simulink model "VTOL_v2_MW"  (R2018b)
settings: Solver=FixedStepAuto  StartTime=0.0  StopTime=inf  FixedStep=Ts  RelTol=1e-3  EnableMultiTasking=on
values from neighbouring files (symbols this model uses):
  Ts = 1/100    (= 0.01)    [VTOL_params.m]
undefined symbols (not defined in the file or in its folder): color, deltaprops, dev, led_mask, Main, mode, MRC, pwm_output0
libraries: aerolibutil x7, px4uORBlib x6, pwm_sig_converters x4, px4Sensorslib x3, simulink x3, px4lib x1, sharedtransform x1
(part 2 of 2)

== matlab function VTOL_v2_MW/PX4 SD Card Logger4/SDCard_logger ==
  data: en input boolean; data input; logname parameter uint8; cacheflag parameter boolean; numRecs parameter uint32
%% PX4 SD Card Logger
% Note: All data needs to be of the same type (e.g. double)
% Header information format:
%           String "MWLOG"
%           Time/Date 4 bytes (time())
%           Number of Signals per record Logged 1 byte (256 max)
%           Data Type of Signals Logged  1 byte (1-10)
%           Number of bytes per record 2 bytes (65535 max)
% This does NOT include the number of data sets logged.
% i.e. The Reader is responsible for reading until EOF.
% Steve Kuznicki
% Copyright 2018 The MathWorks, Inc.

function SDCard_logger(en, data, logname, cacheflag, numRecs)

persistent fp count elem_size vect_size datastore timestore count_prev

if coder.target('Rtw')
    
    coder.cinclude('<stdio.h>');
    coder.cinclude('<time.h>');
    
    if coder.target('Rtw')
        coder.cinclude('<drivers/drv_hrt.h>');
    end
    
    if coder.target('Rtw')
        timestamp=coder.opaque('uint64_t');
        timestamp=coder.ceval('hrt_absolute_time');
    else
        timestamp = uint64(0);
    end
    
    if isempty(count)
        count = uint32(0);
        count_prev=count;
        fp = coder.opaque('FILE*', 'NULL');
        if cacheflag == true
            datastore = zeros(numRecs*uint32(coder.const(numel(data))), 1, 'like', data);
            timestore=uint64(zeros(numRecs, 1));
        end
        
        [elsize, eltype] = get_elem_size(data);
        elem_size = coder.const(uint16(elsize));
        elem_type = coder.const(uint8(eltype));
        vect_size = coder.const(uint8(numel(data)));
        coder.ceval('printf',['OPENING file %s vect_size %d elem_size %d numRecs %d %c' uint8(0)], ...
            [logname,'.bin', int8(0)], uint32(vect_size), uint32(elem_size), uint32(numRecs), uint8(10));
        fp = coder.ceval('fopen', [logname,'.bin', int8(0)], ['wb', int8(0)]);
        
        % Write header information here
        % header token + version
        mlStrVer = 'MWLOG';
        coder.ceval('fwrite', coder.rref(mlStrVer), uint32(1), length(mlStrVer), fp);
        % date/time
        tm = uint32(0);
        tmptr = uint32(0);
        tm = coder.ceval('time',coder.wref(tmptr));
        coder.ceval('fwrite', coder.rref(tm), uint32(4), uint32(1), fp);
        % number of elements in each record
        coder.ceval('fwrite', coder.rref(vect_size), uint32(1), uint32(1), fp);
        % data type of the elements
        coder.ceval('fwrite', coder.rref(elem_type), uint32(1), uint32(1), fp);
        % size of each record in bytes
        recSize = elem_size * uint16(vect_size);
        coder.ceval('fwrite', coder.rref(recSize), uint32(2), uint32(1), fp);
        coder.ceval('fclose', fp);
    end
    
    
    if (en && (count < numRecs))
              
        % cache data in memory or use fwrite
        if cacheflag == true
            addr = (count*uint32(vect_size))+1;
            for idx = 1:vect_size
                datastore(addr) = data(idx);
                addr = addr + 1;
            end
            timestore(count+uint32(1))=uint64(timestamp);
        else
            % open file in append mode
            fp = coder.ceval('fopen', [logname,'.bin', int8(0)], ['ab', int8(0)]);
            coder.ceval('fwrite', coder.rref(data), elem_size, vect_size, fp);
            if coder.target('Rtw')
                coder.ceval('fwrite', coder.rref(timestamp), uint32(8), uint32(1), fp);
            end
            coder.ceval('fflush', fp);
            coder.ceval('fclose', fp);
        end
        count = count + uint32(1);
        
    else
        
        if cacheflag
            % open file in append mode
            fp = coder.ceval('fopen', [logname,'.bin', int8(0)], ['ab', int8(0)]);
            coder.ceval('printf',['CLOSING file. count = %d %c' uint8(0)], uint32(count), uint8(10));
            for idx=count_prev+1:count
                for idx2=(idx-1)*double(vect_size)+1:(idx-1)*double(vect_size)+double(vect_size)
                    coder.ceval('fwrite', coder.rref(datastore(idx2)), elem_size, uint32(1), fp);
                end
                coder.ceval('fwrite', coder.rref(timestore(idx)), uint32(8), uint32(1), fp);
            end
            coder.ceval('fflush', fp);
            coder.ceval('fclose', fp);
        end
        count_prev=count;
    end
end

% return the size of the element in bytes
    function [elem_size, dtype] = get_elem_size(data)
        switch(class(data))
            case 'double'
                elem_size = 8;
                dtype = 1;
            case 'single'
                elem_size = 4;
                dtype = 2;
            case 'int32'
                elem_size = 4;
                dtype = 3;
            case 'uint32'
                elem_size = 4;
                dtype = 4;
            case 'int16'
                elem_size = 2;
                dtype = 5;
            case 'uint16'
                elem_size = 2;
                dtype = 6;
            case 'int8'
                elem_size = 1;
                dtype = 7;
            case 'uint8'
                elem_size = 1;
                dtype = 8;
            case 'logical'
                elem_size = 1;
                dtype = 9;
            case 'embedded.fi'
                nt = numerictype(data);
                elem_size = 2^ceil(log2(ceil(nt.WordLength / 8)));
                dtype = 10;
        end
        if ~isreal(data)
            elem_size = elem_size*2;
        end
        
        elem_size = uint16(elem_size);
        dtype = uint8(dtype);
    end
end

== matlab function VTOL_v2_MW/MATLAB Function12 ==
  data: sticks input; q_ref output; offset_stick input
function q_ref = sticks2quat(sticks, offset_stick)

persistent ail;
persistent ele;
persistent rud;
persistent S2;
if isempty(ail)
    ail = single(0);
end
if isempty(ele)
    ele = single(0);
end
if isempty(rud)
    rud = single(0);
end
if isempty(S2)
    S2 = single(0);
end

offset = 0;

SB = sticks(5); % MOde selector
if SB < -0.1
    % mode hover stable
    %thrust = sticks(1);
    ail = 1.5*sticks(2);
    ele = 1.5*sticks(3);
    rud = 1.5*sticks(4);
    
%elseif SB < 0.1
%    % Not used now
else
    % Mode servo setting quat, acro?
    S2 = 0.05*(sticks(6)+1); % Sensitivity setting
    ail = ail + S2*sticks(2);
    ele = ele + S2*sticks(3);
    rud = rud + S2*sticks(4);
    
end

%ElevonL = -ail-ele;
%ElevonR = -ail+ele;
%ThrustL = thrust+rud;
%ThrustR = thrust-rud;
%{
q_init = [cos(pi/4), 0, sin(pi/4), 0];
qyaw = [q00 0 0 q03];
qpitch = [q10 0 q12 0];
qroll = [q20 q21 0 0];
q0 = quatmultiply(q_init,qyaw)
q1 = quatmultiply(q0, qpitch);
q_ref = quatmultiply(q1,qroll)'
%}

%offset = 0; %deg2rad(5); % set on elevons instead
SA = sticks(7);
if SA < -0.1 % point up for hover
    q_init = [cos((pi/4 + offset)), 0, sin((pi/4 + offset)), 0];
elseif SA < 0.1 % Point forward for flight
    q_init = [cos((pi/20 + offset)), 0, sin((pi/20 + offset)), 0];
else % Point backwards for upsidedown flying
    q_init = [cos((pi/2 + offset)), 0, sin((pi/2 + offset)), 0];
end

q00 = cos(rud/2);
q03 = sin(rud/2);
q10 = cos(-ele/2);
q12 = sin(-ele/2);
q20 = cos(ail/2);
q21 = sin(ail/2);


qyaw = [q00 0 0 q03];
qpitch = [q10 0 q12 0];
qroll = [q20 q21 0 0];

%{
q0 = quatmultiply(qyaw,qpitch);
q1 = quatmultiply(q0, qroll);
q_ref = quatmultiply(q1,q_init)';
 %}
q0 = quatmultiply(q_init, qyaw);
q1 = quatmultiply(q0, qpitch);
q_ref = quatmultiply(q1,qroll)';

== matlab function VTOL_v2_MW/PX4 SD Card Logger1/SDCard_logger ==
  data: en input boolean; data input; logname parameter uint8; cacheflag parameter boolean; numRecs parameter uint32
%% PX4 SD Card Logger
% Note: All data needs to be of the same type (e.g. double)
% Header information format:
%           String "MWLOG"
%           Time/Date 4 bytes (time())
%           Number of Signals per record Logged 1 byte (256 max)
%           Data Type of Signals Logged  1 byte (1-10)
%           Number of bytes per record 2 bytes (65535 max)
% This does NOT include the number of data sets logged.
% i.e. The Reader is responsible for reading until EOF.
% Steve Kuznicki
% Copyright 2018 The MathWorks, Inc.

function SDCard_logger(en, data, logname, cacheflag, numRecs)

persistent fp count elem_size vect_size datastore timestore count_prev

if coder.target('Rtw')
    
    coder.cinclude('<stdio.h>');
    coder.cinclude('<time.h>');
    
    if coder.target('Rtw')
        coder.cinclude('<drivers/drv_hrt.h>');
    end
    
    if coder.target('Rtw')
        timestamp=coder.opaque('uint64_t');
        timestamp=coder.ceval('hrt_absolute_time');
    else
        timestamp = uint64(0);
    end
    
    if isempty(count)
        count = uint32(0);
        count_prev=count;
        fp = coder.opaque('FILE*', 'NULL');
        if cacheflag == true
            datastore = zeros(numRecs*uint32(coder.const(numel(data))), 1, 'like', data);
            timestore=uint64(zeros(numRecs, 1));
        end
        
        [elsize, eltype] = get_elem_size(data);
        elem_size = coder.const(uint16(elsize));
        elem_type = coder.const(uint8(eltype));
        vect_size = coder.const(uint8(numel(data)));
        coder.ceval('printf',['OPENING file %s vect_size %d elem_size %d numRecs %d %c' uint8(0)], ...
            [logname,'.bin', int8(0)], uint32(vect_size), uint32(elem_size), uint32(numRecs), uint8(10));
        fp = coder.ceval('fopen', [logname,'.bin', int8(0)], ['wb', int8(0)]);
        
        % Write header information here
        % header token + version
        mlStrVer = 'MWLOG';
        coder.ceval('fwrite', coder.rref(mlStrVer), uint32(1), length(mlStrVer), fp);
        % date/time
        tm = uint32(0);
        tmptr = uint32(0);
        tm = coder.ceval('time',coder.wref(tmptr));
        coder.ceval('fwrite', coder.rref(tm), uint32(4), uint32(1), fp);
        % number of elements in each record
        coder.ceval('fwrite', coder.rref(vect_size), uint32(1), uint32(1), fp);
        % data type of the elements
        coder.ceval('fwrite', coder.rref(elem_type), uint32(1), uint32(1), fp);
        % size of each record in bytes
        recSize = elem_size * uint16(vect_size);
        coder.ceval('fwrite', coder.rref(recSize), uint32(2), uint32(1), fp);
        coder.ceval('fclose', fp);
    end
    
    
    if (en && (count < numRecs))
              
        % cache data in memory or use fwrite
        if cacheflag == true
            addr = (count*uint32(vect_size))+1;
            for idx = 1:vect_size
                datastore(addr) = data(idx);
                addr = addr + 1;
            end
            timestore(count+uint32(1))=uint64(timestamp);
        else
            % open file in append mode
            fp = coder.ceval('fopen', [logname,'.bin', int8(0)], ['ab', int8(0)]);
            coder.ceval('fwrite', coder.rref(data), elem_size, vect_size, fp);
            if coder.target('Rtw')
                coder.ceval('fwrite', coder.rref(timestamp), uint32(8), uint32(1), fp);
            end
            coder.ceval('fflush', fp);
            coder.ceval('fclose', fp);
        end
        count = count + uint32(1);
        
   else
        
        if cacheflag
            % open file in append mode
            fp = coder.ceval('fopen', [logname,'.bin', int8(0)], ['ab', int8(0)]);
            coder.ceval('printf',['CLOSING file. count = %d %c' uint8(0)], uint32(count), uint8(10));
            for idx=count_prev+1:count
                for idx2=(idx-1)*double(vect_size)+1:(idx-1)*double(vect_size)+double(vect_size)
                    coder.ceval('fwrite', coder.rref(datastore(idx2)), elem_size, uint32(1), fp);
                end
                coder.ceval('fwrite', coder.rref(timestore(idx)), uint32(8), uint32(1), fp);
            end
            coder.ceval('fflush', fp);
            coder.ceval('fclose', fp);
        end
        count_prev=count;
    end
end

% return the size of the element in bytes
    function [elem_size, dtype] = get_elem_size(data)
        switch(class(data))
            case 'double'
                elem_size = 8;
                dtype = 1;
            case 'single'
                elem_size = 4;
                dtype = 2;
            case 'int32'
                elem_size = 4;
                dtype = 3;
            case 'uint32'
                elem_size = 4;
                dtype = 4;
            case 'int16'
                elem_size = 2;
                dtype = 5;
            case 'uint16'
                elem_size = 2;
                dtype = 6;
            case 'int8'
                elem_size = 1;
                dtype = 7;
            case 'uint8'
                elem_size = 1;
                dtype = 8;
            case 'logical'
                elem_size = 1;
                dtype = 9;
            case 'embedded.fi'
                nt = numerictype(data);
                elem_size = 2^ceil(log2(ceil(nt.WordLength / 8)));
                dtype = 10;
        end
        if ~isreal(data)
            elem_size = elem_size*2;
        end
        
        elem_size = uint16(elem_size);
        dtype = uint8(dtype);
    end
end

== matlab function VTOL_v2_MW/Subsystem/MATLAB Function14 ==
  data: target_altitude output single; throttle input single; init_alt input single
function target_altitude = fcn(throttle, init_alt)

persistent target_alt;
if isempty(target_alt)
    target_alt = init_alt;
end

target_alt = target_alt + 0.005*throttle;
target_altitude = target_alt;

== matlab function VTOL_v2_MW/MATLAB Function14 ==
  data: tao input; u_deltaL output; u_omegaL input; u_omegaR input; v input; u_deltaR output
function [u_deltaL, u_deltaR] = torqueConverter(tao, u_omegaL, u_omegaR, v)

KV = 1300;
V = 3.7*3;
loadFactor = 0.5;
maxRPM = KV*V*loadFactor;

omegaL = maxRPM*0.5*(u_omegaL+1); % Shift from [-1,1] to [0,1]
omegaR = maxRPM*0.5*(u_omegaR+1);
k1 = 0;
k2 = 2.41e-6;
k3 = 0;
k4 = 4.06e-6;

% These functons are derived in my paper, see
% https://github.com/Trobolit/MastersThesis/blob/master/thesis/main.pdf
u_deltaL = -0.5*tao(2)/(k1*sign(v(1))*sum(v.^2) + k2*omegaL^2) ...
           - 0.5*tao(1)/(k3*sign(v(1))*sum(v.^2) + k4*omegaL^2);

u_deltaR = -0.5*tao(2)/(k1*sign(v(1))*sum(v.^2) + k2*omegaR^2) ...
           + 0.5*tao(1)/(k3*sign(v(1))*sum(v.^2) + k4*omegaR^2);

== matlab function VTOL_v2_MW/MATLAB Function11 ==
  data: P input; D input; axisgains input; angErr input; taos output; w input
function taos = taos_fordecoupler(P, D, axisgains,angErr, w)

taos = single([0;0;0]);

%P1 = 1; %30; %1
%P2 = 0.5; %7.5; %0.25
cx = axisgains(1);%10;
cy = axisgains(2);%100;
cz = axisgains(3);%1;


% Emil Fresk P2 controller
taos = -P.*angErr - D.*w;
% Adjustment for actuators
taos(1) = cx*taos(1);
taos(2) = cy*taos(2);
taos(3) = cz*taos(3);

== matlab function VTOL_v2_MW/MATLAB Function15 ==
  data: voltage input single; stopsig output uint16; cutoff input single
function stopsig = fcn(voltage, cutoff)

if voltage<cutoff
    stopsig = uint16(2000);
else
    stopsig = uint16(1000);
end

== matlab function VTOL_v2_MW/MATLAB Function16 ==
  data: offset_stick input; offset output
function offset = fcn(offset_stick)

offset = single(offset_stick);
% Shift to center
offset = offset-1500;
% Range is ~1000-2000, ie +-500, but in is +-1
offset = 0.5*offset./500 + 0.75;

== matlab function VTOL_v2_MW/PX4 SD Card Logger3/SDCard_logger ==
  data: en input boolean; data input; logname parameter uint8; cacheflag parameter boolean; numRecs parameter uint32
%% PX4 SD Card Logger
% Note: All data needs to be of the same type (e.g. double)
% Header information format:
%           String "MWLOG"
%           Time/Date 4 bytes (time())
%           Number of Signals per record Logged 1 byte (256 max)
%           Data Type of Signals Logged  1 byte (1-10)
%           Number of bytes per record 2 bytes (65535 max)
% This does NOT include the number of data sets logged.
% i.e. The Reader is responsible for reading until EOF.
% Steve Kuznicki
% Copyright 2018 The MathWorks, Inc.

function SDCard_logger(en, data, logname, cacheflag, numRecs)

persistent fp count elem_size vect_size datastore timestore count_prev

if coder.target('Rtw')
    
    coder.cinclude('<stdio.h>');
    coder.cinclude('<time.h>');
    
    if coder.target('Rtw')
        coder.cinclude('<drivers/drv_hrt.h>');
    end
    
    if coder.target('Rtw')
        timestamp=coder.opaque('uint64_t');
        timestamp=coder.ceval('hrt_absolute_time');
    else
        timestamp = uint64(0);
    end
    
    if isempty(count)
        count = uint32(0);
        count_prev=count;
        fp = coder.opaque('FILE*', 'NULL');
        if cacheflag == true
            datastore = zeros(numRecs*uint32(coder.const(numel(data))), 1, 'like', data);
            timestore=uint64(zeros(numRecs, 1));
        end
        
        [elsize, eltype] = get_elem_size(data);
        elem_size = coder.const(uint16(elsize));
        elem_type = coder.const(uint8(eltype));
        vect_size = coder.const(uint8(numel(data)));
        coder.ceval('printf',['OPENING file %s vect_size %d elem_size %d numRecs %d %c' uint8(0)], ...
            [logname,'.bin', int8(0)], uint32(vect_size), uint32(elem_size), uint32(numRecs), uint8(10));
        fp = coder.ceval('fopen', [logname,'.bin', int8(0)], ['wb', int8(0)]);
        
        % Write header information here
        % header token + version
        mlStrVer = 'MWLOG';
        coder.ceval('fwrite', coder.rref(mlStrVer), uint32(1), length(mlStrVer), fp);
        % date/time
        tm = uint32(0);
        tmptr = uint32(0);
        tm = coder.ceval('time',coder.wref(tmptr));
        coder.ceval('fwrite', coder.rref(tm), uint32(4), uint32(1), fp);
        % number of elements in each record
        coder.ceval('fwrite', coder.rref(vect_size), uint32(1), uint32(1), fp);
        % data type of the elements
        coder.ceval('fwrite', coder.rref(elem_type), uint32(1), uint32(1), fp);
        % size of each record in bytes
        recSize = elem_size * uint16(vect_size);
        coder.ceval('fwrite', coder.rref(recSize), uint32(2), uint32(1), fp);
        coder.ceval('fclose', fp);
    end
    
    
    if (en && (count < numRecs))
              
        % cache data in memory or use fwrite
        if cacheflag == true
            addr = (count*uint32(vect_size))+1;
            for idx = 1:vect_size
                datastore(addr) = data(idx);
                addr = addr + 1;
            end
            timestore(count+uint32(1))=uint64(timestamp);
        else
            % open file in append mode
            fp = coder.ceval('fopen', [logname,'.bin', int8(0)], ['ab', int8(0)]);
            coder.ceval('fwrite', coder.rref(data), elem_size, vect_size, fp);
            if coder.target('Rtw')
                coder.ceval('fwrite', coder.rref(timestamp), uint32(8), uint32(1), fp);
            end
            coder.ceval('fflush', fp);
            coder.ceval('fclose', fp);
        end
        count = count + uint32(1);
        
    else
        
        if cacheflag
            % open file in append mode
            fp = coder.ceval('fopen', [logname,'.bin', int8(0)], ['ab', int8(0)]);
            coder.ceval('printf',['CLOSING file. count = %d %c' uint8(0)], uint32(count), uint8(10));
            for idx=count_prev+1:count
                for idx2=(idx-1)*double(vect_size)+1:(idx-1)*double(vect_size)+double(vect_size)
                    coder.ceval('fwrite', coder.rref(datastore(idx2)), elem_size, uint32(1), fp);
                end
                coder.ceval('fwrite', coder.rref(timestore(idx)), uint32(8), uint32(1), fp);
            end
            coder.ceval('fflush', fp);
            coder.ceval('fclose', fp);
        end
        count_prev=count;
    end
end

% return the size of the element in bytes
    function [elem_size, dtype] = get_elem_size(data)
        switch(class(data))
            case 'double'
                elem_size = 8;
                dtype = 1;
            case 'single'
                elem_size = 4;
                dtype = 2;
            case 'int32'
                elem_size = 4;
                dtype = 3;
            case 'uint32'
                elem_size = 4;
                dtype = 4;
            case 'int16'
                elem_size = 2;
                dtype = 5;
            case 'uint16'
                elem_size = 2;
                dtype = 6;
            case 'int8'
                elem_size = 1;
                dtype = 7;
            case 'uint8'
                elem_size = 1;
                dtype = 8;
            case 'logical'
                elem_size = 1;
                dtype = 9;
            case 'embedded.fi'
                nt = numerictype(data);
                elem_size = 2^ceil(log2(ceil(nt.WordLength / 8)));
                dtype = 10;
        end
        if ~isreal(data)
            elem_size = elem_size*2;
        end
        
        elem_size = uint16(elem_size);
        dtype = uint8(dtype);
    end
end

== matlab function VTOL_v2_MW/TorqueTranslator ==
  data: u_jointT input; states input; wdots input; pitchoffset input; u_omegaL output; u_omegaR output; u_deltaL output; u_deltaR output
function [u_omegaL, u_omegaR, u_deltaL, u_deltaR] = torqueConverter(u_jointT,states, wdots, pitchoffset)

% The reference coming in is for angular accelleration, so don't treat it
% as pure torque:
% I*wdot = tao 

%wxr = taos(1)./p.Ix; 
%wyr = taos(2)./p.Iy;
%wzr = taos(3)./p.Iz;

Ix=single(0.07/4); % kg*m^2
Iy=single(0.0079/4);
Iz=single(0.08/4);
tx = wdots(1)*Ix;
ty = wdots(2)*Iy;
tz = wdots(3)*Iz;

omegaL = states(13);
omegaR = states(14);

%init outputs
u_deltaL = 0;
u_deltaR = 0;
u_omegaL = 0;
u_omegaR = 0;


% We assume propellers always spin one way. Never reverse.
% We know wanted torque, i.e. we know wdot*Iz=taoz=p.yt*(TL-TR)=p.yt*dT
yt = single(0.33);
K_T = single(3.0488e-05);
u_omegaL2 = (u_jointT+(tz/yt)/2)/K_T ; % THese share the jointT, half each.
u_omegaR2 =  (u_jointT-(tz/yt)/2)/K_T ;
if u_omegaL2 < 0
    u_omegaL = single(0);
else
    u_omegaL = sqrt(u_omegaL2);
end
if u_omegaR2 < 0
    u_omegaR = single(0);
else
    u_omegaR = sqrt(u_omegaR2);
end

% Lets make a few (crude) approximations.
% - Damping due to rotational speed doesn't exist.
% - Winglets have no z-offset.
% - Wings provide no pitch moment from lift
% Then we come to these formulas for torque around each axis:
%f1 = p.yf.*(FLT+FL -FRT-FR)
%f2 = p.xf.*(FLT+FL+FRT+FR) ...
%f3 = p.yt.*(TL-TR) ...
% 
% They essentially say that aileroins are effective proportioanlly to the
% (square) of the air velocity over them.
% Lets invert that and use as our tunable gain.

%{
% airflow in thrust wake
b_w = 0.01;
v_w_L = b_w .* omegaL; %[b_w .* omegaL; vy; vz];
v_w_R = b_w .* omegaR;
% AILERONS
% Lift inside wake, signs bc rotation dir of aileron
%dFT = -p.CLdelta * 0.5*p.rho * p.Saw;% * deltaL*v_w_L.^2;
rho = 1.225;
Saw = 0.0091;
 dFT = -0.5*rho * Saw;% * deltaR*v_w_R.^2;
%}

% Below only includes sensitivity from airflow % The pitch offet is our
% mechanical trim on the aircraft.
omegaL_f = omegaL; %omegas_filt(1);
omegaR_f = omegaR; %omegas_filt(2);
u_deltaL = -ty / ( 2*2.41e-6*omegaL_f.^2) - tx / (2*4.06e-6*omegaL_f.^2) + pitchoffset;
u_deltaR =  tx / ( 2*4.06e-6*omegaR_f.^2) - ty / (2*2.41e-6*omegaR_f.^2) + pitchoffset;

== matlab function VTOL_v2_MW/PX4 SD Card Logger5/SDCard_logger ==
  data: en input boolean; data input; logname parameter uint8; cacheflag parameter boolean; numRecs parameter uint32
%% PX4 SD Card Logger
% Note: All data needs to be of the same type (e.g. double)
% Header information format:
%           String "MWLOG"
%           Time/Date 4 bytes (time())
%           Number of Signals per record Logged 1 byte (256 max)
%           Data Type of Signals Logged  1 byte (1-10)
%           Number of bytes per record 2 bytes (65535 max)
% This does NOT include the number of data sets logged.
% i.e. The Reader is responsible for reading until EOF.
% Steve Kuznicki
% Copyright 2018 The MathWorks, Inc.

function SDCard_logger(en, data, logname, cacheflag, numRecs)

persistent fp count elem_size vect_size datastore timestore count_prev

if coder.target('Rtw')
    
    coder.cinclude('<stdio.h>');
    coder.cinclude('<time.h>');
    
    if coder.target('Rtw')
        coder.cinclude('<drivers/drv_hrt.h>');
    end
    
    if coder.target('Rtw')
        timestamp=coder.opaque('uint64_t');
        timestamp=coder.ceval('hrt_absolute_time');
    else
        timestamp = uint64(0);
    end
    
    if isempty(count)
        count = uint32(0);
        count_prev=count;
        fp = coder.opaque('FILE*', 'NULL');
        if cacheflag == true
            datastore = zeros(numRecs*uint32(coder.const(numel(data))), 1, 'like', data);
            timestore=uint64(zeros(numRecs, 1));
        end
        
        [elsize, eltype] = get_elem_size(data);
        elem_size = coder.const(uint16(elsize));
        elem_type = coder.const(uint8(eltype));
        vect_size = coder.const(uint8(numel(data)));
        coder.ceval('printf',['OPENING file %s vect_size %d elem_size %d numRecs %d %c' uint8(0)], ...
            [logname,'.bin', int8(0)], uint32(vect_size), uint32(elem_size), uint32(numRecs), uint8(10));
        fp = coder.ceval('fopen', [logname,'.bin', int8(0)], ['wb', int8(0)]);
        
        % Write header information here
        % header token + version
        mlStrVer = 'MWLOG';
        coder.ceval('fwrite', coder.rref(mlStrVer), uint32(1), length(mlStrVer), fp);
        % date/time
        tm = uint32(0);
        tmptr = uint32(0);
        tm = coder.ceval('time',coder.wref(tmptr));
        coder.ceval('fwrite', coder.rref(tm), uint32(4), uint32(1), fp);
        % number of elements in each record
        coder.ceval('fwrite', coder.rref(vect_size), uint32(1), uint32(1), fp);
        % data type of the elements
        coder.ceval('fwrite', coder.rref(elem_type), uint32(1), uint32(1), fp);
        % size of each record in bytes
        recSize = elem_size * uint16(vect_size);
        coder.ceval('fwrite', coder.rref(recSize), uint32(2), uint32(1), fp);
        coder.ceval('fclose', fp);
    end
    
    
    if (en && (count < numRecs))
              
        % cache data in memory or use fwrite
        if cacheflag == true
            addr = (count*uint32(vect_size))+1;
            for idx = 1:vect_size
                datastore(addr) = data(idx);
                addr = addr + 1;
            end
            timestore(count+uint32(1))=uint64(timestamp);
        else
            % open file in append mode
            fp = coder.ceval('fopen', [logname,'.bin', int8(0)], ['ab', int8(0)]);
            coder.ceval('fwrite', coder.rref(data), elem_size, vect_size, fp);
            if coder.target('Rtw')
                coder.ceval('fwrite', coder.rref(timestamp), uint32(8), uint32(1), fp);
            end
            coder.ceval('fflush', fp);
            coder.ceval('fclose', fp);
        end
        count = count + uint32(1);
        
    else
        
        if cacheflag
            % open file in append mode
            fp = coder.ceval('fopen', [logname,'.bin', int8(0)], ['ab', int8(0)]);
            coder.ceval('printf',['CLOSING file. count = %d %c' uint8(0)], uint32(count), uint8(10));
            for idx=count_prev+1:count
                for idx2=(idx-1)*double(vect_size)+1:(idx-1)*double(vect_size)+double(vect_size)
                    coder.ceval('fwrite', coder.rref(datastore(idx2)), elem_size, uint32(1), fp);
                end
                coder.ceval('fwrite', coder.rref(timestore(idx)), uint32(8), uint32(1), fp);
            end
            coder.ceval('fflush', fp);
            coder.ceval('fclose', fp);
        end
        count_prev=count;
    end
end

% return the size of the element in bytes
    function [elem_size, dtype] = get_elem_size(data)
        switch(class(data))
            case 'double'
                elem_size = 8;
                dtype = 1;
            case 'single'
                elem_size = 4;
                dtype = 2;
            case 'int32'
                elem_size = 4;
                dtype = 3;
            case 'uint32'
                elem_size = 4;
                dtype = 4;
            case 'int16'
                elem_size = 2;
                dtype = 5;
            case 'uint16'
                elem_size = 2;
                dtype = 6;
            case 'int8'
                elem_size = 1;
                dtype = 7;
            case 'uint8'
                elem_size = 1;
                dtype = 8;
            case 'logical'
                elem_size = 1;
                dtype = 9;
            case 'embedded.fi'
                nt = numerictype(data);
                elem_size = 2^ceil(log2(ceil(nt.WordLength / 8)));
                dtype = 10;
        end
        if ~isreal(data)
            elem_size = elem_size*2;
        end
        
        elem_size = uint16(elem_size);
        dtype = uint8(dtype);
    end
end

== matlab function VTOL_v2_MW/MATLAB Function17 ==
  data: u input; y output
function y = logstarter(u)
%At first arm, start logging and dont quit

persistent state;

if isempty(state)
    state = 0;
end

if u>0
    state = 1;
end

y = state;

== matlab function VTOL_v2_MW/PX4 SD Card Logger6/SDCard_logger ==
  data: en input boolean; data input; logname parameter uint8; cacheflag parameter boolean; numRecs parameter uint32
%% PX4 SD Card Logger
% Note: All data needs to be of the same type (e.g. double)
% Header information format:
%           String "MWLOG"
%           Time/Date 4 bytes (time())
%           Number of Signals per record Logged 1 byte (256 max)
%           Data Type of Signals Logged  1 byte (1-10)
%           Number of bytes per record 2 bytes (65535 max)
% This does NOT include the number of data sets logged.
% i.e. The Reader is responsible for reading until EOF.
% Steve Kuznicki
% Copyright 2018 The MathWorks, Inc.

function SDCard_logger(en, data, logname, cacheflag, numRecs)

persistent fp count elem_size vect_size datastore timestore count_prev

if coder.target('Rtw')
    
    coder.cinclude('<stdio.h>');
    coder.cinclude('<time.h>');
    
    if coder.target('Rtw')
        coder.cinclude('<drivers/drv_hrt.h>');
    end
    
    if coder.target('Rtw')
        timestamp=coder.opaque('uint64_t');
        timestamp=coder.ceval('hrt_absolute_time');
    else
        timestamp = uint64(0);
    end
    
    if isempty(count)
        count = uint32(0);
        count_prev=count;
        fp = coder.opaque('FILE*', 'NULL');
        if cacheflag == true
            datastore = zeros(numRecs*uint32(coder.const(numel(data))), 1, 'like', data);
            timestore=uint64(zeros(numRecs, 1));
        end
        
        [elsize, eltype] = get_elem_size(data);
        elem_size = coder.const(uint16(elsize));
        elem_type = coder.const(uint8(eltype));
        vect_size = coder.const(uint8(numel(data)));
        coder.ceval('printf',['OPENING file %s vect_size %d elem_size %d numRecs %d %c' uint8(0)], ...
            [logname,'.bin', int8(0)], uint32(vect_size), uint32(elem_size), uint32(numRecs), uint8(10));
        fp = coder.ceval('fopen', [logname,'.bin', int8(0)], ['wb', int8(0)]);
        
        % Write header information here
        % header token + version
        mlStrVer = 'MWLOG';
        coder.ceval('fwrite', coder.rref(mlStrVer), uint32(1), length(mlStrVer), fp);
        % date/time
        tm = uint32(0);
        tmptr = uint32(0);
        tm = coder.ceval('time',coder.wref(tmptr));
        coder.ceval('fwrite', coder.rref(tm), uint32(4), uint32(1), fp);
        % number of elements in each record
        coder.ceval('fwrite', coder.rref(vect_size), uint32(1), uint32(1), fp);
        % data type of the elements
        coder.ceval('fwrite', coder.rref(elem_type), uint32(1), uint32(1), fp);
        % size of each record in bytes
        recSize = elem_size * uint16(vect_size);
        coder.ceval('fwrite', coder.rref(recSize), uint32(2), uint32(1), fp);
        coder.ceval('fclose', fp);
    end
    
    
    if (en && (count < numRecs))
              
        % cache data in memory or use fwrite
        if cacheflag == true
            addr = (count*uint32(vect_size))+1;
            for idx = 1:vect_size
                datastore(addr) = data(idx);
                addr = addr + 1;
            end
            timestore(count+uint32(1))=uint64(timestamp);
        else
            % open file in append mode
            fp = coder.ceval('fopen', [logname,'.bin', int8(0)], ['ab', int8(0)]);
            coder.ceval('fwrite', coder.rref(data), elem_size, vect_size, fp);
            if coder.target('Rtw')
                coder.ceval('fwrite', coder.rref(timestamp), uint32(8), uint32(1), fp);
            end
            coder.ceval('fflush', fp);
            coder.ceval('fclose', fp);
        end
        count = count + uint32(1);
        
    else
        
        if cacheflag
            % open file in append mode
            fp = coder.ceval('fopen', [logname,'.bin', int8(0)], ['ab', int8(0)]);
            coder.ceval('printf',['CLOSING file. count = %d %c' uint8(0)], uint32(count), uint8(10));
            for idx=count_prev+1:count
                for idx2=(idx-1)*double(vect_size)+1:(idx-1)*double(vect_size)+double(vect_size)
                    coder.ceval('fwrite', coder.rref(datastore(idx2)), elem_size, uint32(1), fp);
                end
                coder.ceval('fwrite', coder.rref(timestore(idx)), uint32(8), uint32(1), fp);
            end
            coder.ceval('fflush', fp);
            coder.ceval('fclose', fp);
        end
        count_prev=count;
    end
end

% return the size of the element in bytes
    function [elem_size, dtype] = get_elem_size(data)
        switch(class(data))
            case 'double'
                elem_size = 8;
                dtype = 1;
            case 'single'
                elem_size = 4;
                dtype = 2;
            case 'int32'
                elem_size = 4;
                dtype = 3;
            case 'uint32'
                elem_size = 4;
                dtype = 4;
            case 'int16'
                elem_size = 2;
                dtype = 5;
            case 'uint16'
                elem_size = 2;
                dtype = 6;
            case 'int8'
                elem_size = 1;
                dtype = 7;
            case 'uint8'
                elem_size = 1;
                dtype = 8;
            case 'logical'
                elem_size = 1;
                dtype = 9;
            case 'embedded.fi'
                nt = numerictype(data);
                elem_size = 2^ceil(log2(ceil(nt.WordLength / 8)));
                dtype = 10;
        end
        if ~isreal(data)
            elem_size = elem_size*2;
        end
        
        elem_size = uint16(elem_size);
        dtype = uint8(dtype);
    end
end

== matlab function VTOL_v2_MW/MATLAB Function18 ==
  data: u input; y output
function y = fcn(u)

if u>uint16(1300)
    y = logical(true);
else
    y = logical(false);
end
